simulink model "bai30"  (R2016a)
settings: Solver=VariableStepAuto  StartTime=0.0  StopTime=10.0  RelTol=1e-3
settings Model: Creator=HP  LastModifiedBy=HP

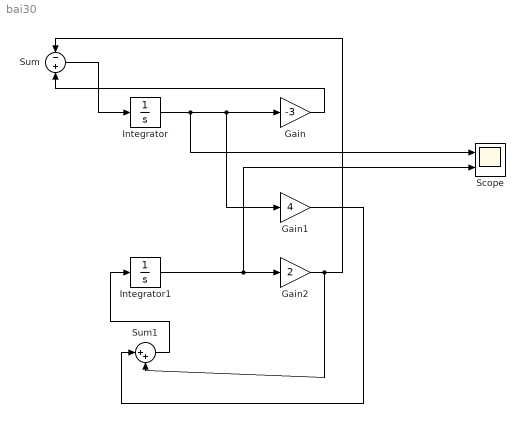
== system bai30 ==
  Gain : Gain  Gain=-3
  Gain1 : Gain  Gain=4
  Gain2 : Gain  Gain=2
  Integrator : Integrator  InitialCondition=1
  Integrator1 : Integrator  InitialCondition=1
  Scope : Scope  NumInputPorts=2
  Sum : Sum  Inputs=-+
  Sum1 : Sum  Inputs=|++
  wires:
  Integrator1/1 -> Scope/2, Gain2/1
  Sum1/1 -> Integrator1/1
  Gain2/1 -> Sum1/2, Sum/1
  Gain1/1 -> Sum1/1
  Gain/1 -> Sum/2
  Sum/1 -> Integrator/1
  Integrator/1 -> Scope/1, Gain1/1, Gain/1
